simulink library "xrbsImage_r4"  (Simulink 7.1)
libraries: xbsIndex_r4 x24, xrbsDSP_r4 x5, xrbsImage_r4 x4
settings Model: Creator=singhj  LastModifiedBy=sysgengroup

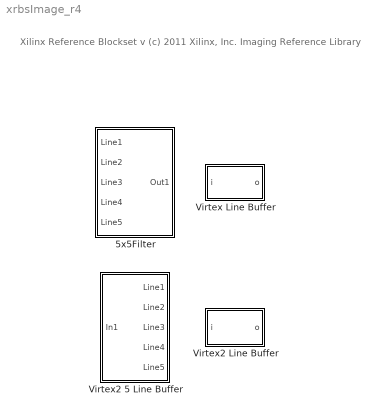
== system xrbsImage_r4 ==
  note: Xilinx Reference Blockset v
      | (c) 2011 Xilinx, Inc.
      |
      | Imaging Reference Library
  5x5Filter : Subsystem  mask(5x5 Filter){maskNum=Edge, coef_n_bits=6, coef_bin_pt=0, smpl_n_bits=8, smpl_bin_pt=0, smpl_period=1, maskVal=0, maskDiv=0}
      mask prompts: maskNum "5x5 Mask"; coef_n_bits "Number of Bits per Coefficient"; coef_bin_pt "Binary Point for Coefficient"; smpl_n_bits "Number of Bits per Input Sample"; smpl_bin_pt "Binary Point for Input Samples"; smpl_period "Sample Period"; maskVal "Mask Value"; maskDiv "Mask Division"
      mask help: The Xilinx 5x5 Filter reference block is implemented using 5 n-tap MAC FIR Filters. Nine different 2-D filters have been provided to filter grayscale images.
      mask init:
      | [bg,fg] = xlcmap('XBlock',0);
      | iPos = get_param(gcb,'Position');
      | iWidth=iPos(3)-iPos(1); iHeight=iPos(4)-iPos(2);
      | iCx=iWidth/2;
      | iCy=iHeight/2;
      | [logoX, logoY] = xlogo(iPos);
      | 
      | % Different 5x5 Filters 
      | %  by default edge is used
      | 
      | edge = [ 0  0  0  0 0; ...
      |          0 -1 -1 -1 0; ...
      |          0 -1  8 -1 0; ...
      |          0 -1 -1 -1 0; ...
      |          0  0  0  0 0];
      | edgeDiv = 1;
      | 
      | sobelX = [ 0  0  0  0 0; ...
      |            0 -1  0  1 0; ...
      |            0 -2  0  2 0; ...
      |            0 -1  0  1 0; ...
      |            0  0  0  0 0];
      | sobelXDiv = 1;
      | 
      | sobelY = [ 0  0  0  0 0; ...
      |            0  1  2  1 0; ...
      |            0  0  0  0 0; ...
      |            0 -1 -2 -1 0; ...
      |            0  0  0  0 0];
      | sobelYDiv = 1;
      | 
      | sobelXY = [ 0  0  0  0 0; ...
      |             0  0 -1 -1 0; ...
      |             0  1  0 -1 0; ...
      |             0  1  1  0 0; ...
      |             0  0  0  0 0];
      | sobelXYDiv = 1;
      | 
      | blur = [ 1  1  1  1 1; ...
      |          1  0  0  0 1; ...
      |          1  0  0  0 1; ...
      |          1  0  0  0 1; ...
      |          1  1  1  1 1];
      | blurDiv = 1/16;
      | 
      | smooth = [ 1  1  1  1 1; ...
      |            1  5  5  5 1; ...
      |            1  5 44  5 1; ...
      |            1  5  5  5 1; ...
      |            1  1  1  1 1];
      | smoothDiv = 1/100;
      | 
      | sharpen = [ 0  0  0  0 0; ...
      |             0 -2 -2 -2 0; ...
      |             0 -2 32 -2 0; ...
      |             0 -2 -2 -2 0; ...
      |             0  0  0  0 0];
      | sharpenDiv = 1/16;
      | 
      | 
      | gaussian = [1 1 2 1 1; ...
      |             1 2 4 2 1; ...
      |             2 4 8 4 2; ...
      |             1 2 4 2 1; ...
      |             1 1 2 1 1];
      | gaussianDiv = 1/52;
      | 
      | identity = [ 0  0  0  0 0; ...
      |              0  0  0  0 0; ...
      |              0  0  1  0 0; ...
      |              0  0  0  0 0; ...
      |              0  0  0  0 0];
      | identityDiv = 1;
      | 
      | maskVal = zeros(5,5,5);
      | maskVal(:,:,1) = edge;
      | maskVal(:,:,2) = sobelX;
      | maskVal(:,:,3) = sobelY;
      | maskVal(:,:,4) = sobelXY;
      | maskVal(:,:,5) = blur;
      | maskVal(:,:,6) = smooth;
      | maskVal(:,:,7) = sharpen;
      | maskVal(:,:,8) = gaussian;
      | maskVal(:,:,9) = identity;
      | 
      | maskDiv = [edgeDiv sobelXDiv sobelYDiv sobelXYDiv blurDiv smoothDiv sharpenDiv gaussianDiv identityDiv];
      mask Help: eval('');xlDoc('-book','sysgen','-topic','x5x5Filter');
      mask StyleString: popup(Edge|Sobel X|Sobel Y|Sobel X-Y|Blur|Smooth|Sharpen|Gaussian|Identity),edit,edit,edit,edit,edit,edit,edit
      mask Display:
      | patch([0 iWidth iWidth 0],[0 0 iHeight iHeight] , bg);
      | patch(logoX,logoY , fg);
      | port_label('input',1,'Line1');
      | port_label('input',2,'Line2');
      | port_label('input',3,'Line3');
      | port_label('input',4,'Line4');
      | port_label('input',5,'Line5');
      | port_label('output',1,'out');
      | plot([0 0 iWidth iWidth 0], [0 iHeight iHeight 0 0]);
  Virtex Line Buffer : Subsystem  mask(Virtex Line Buffer){buf_depth=64, cst=1}
      mask prompts: buf_depth "Buffer Depth"; cst "Sample Period"
      mask help: The Xilinx Virtex Line Buffer reference block delayes a sequential stream of pixels by the specified buffer depth.
      mask init:
      | str = sprintf('-%d',buf_depth);
      | [bg,fg] = xlcmap('XBlock',0);
      | iPos = get_param(gcb,'Position');
      | iWidth=iPos(3)-iPos(1); iHeight=iPos(4)-iPos(2);
      | iCx=iWidth/2;
      | iCy=iHeight/2;
      | [logoX, logoY] = xlogo(iPos);
      mask Help: eval('');xlDoc('-book','sysgen','-topic','Virtex_Line_Buffer');
      mask Display:
      | patch([0 iWidth iWidth 0],[0 0 iHeight iHeight] , bg);
      | patch(logoX,logoY , fg);
      | text(iCx-6,iCy,'z');
      | text(iCx,iCy+4,str);
      | plot([0 0 iWidth iWidth 0], [0 iHeight iHeight 0 0]);
  Virtex2 5 Line Buffer : Subsystem  mask(Virtex2 5 Line Buffer){line_size=64, cst=1}
      mask prompts: line_size "Line Size"; cst "Sample Period"
      mask help: The block buffers a sequential stream of pixels to construct 5 lines of output. Each line is delayed by N samples, where N is the length of the line. Line 1 is delayed 4*N samples, each of the following lines are delay by N fewer samples, and line 5 is a copy of the input.
      mask init:
      | [bg,fg] = xlcmap('XBlock',0);
      | iPos = get_param(gcb,'Position');
      | iWidth=iPos(3)-iPos(1); iHeight=iPos(4)-iPos(2);
      | iCx=iWidth/2;
      | iCy=iHeight/2;
      | [logoX, logoY] = xlogo(iPos);
      mask Help: eval('');xlDoc('-book','sysgen','-topic','Virtex2_5_Line_Buffer');
      mask Display:
      | patch([0 iWidth iWidth 0],[0 0 iHeight iHeight] , bg);
      | patch(logoX,logoY , fg);
      | port_label('input',1,'in');
      | port_label('output',1,'Line1');
      | port_label('output',2,'Line2');
      | port_label('output',3,'Line3');
      | port_label('output',4,'Line4');
      | port_label('output',5,'Line5');
      | plot([0 0 iWidth iWidth 0], [0 iHeight iHeight 0 0]);
  Virtex2 Line Buffer : Subsystem  mask(Virtex2 Line Buffer){buf_depth=64, cst=1}
      mask prompts: buf_depth "Buffer Depth"; cst "Sample Period"
      mask help: The Xilinx Virtex2 Line Buffer reference block delayes a sequential stream of pixels by the specified buffer depth. It is optimized for the Virtex2 family since it uses the Read Before Write option on the underlying Single Port RAM block.
      mask init: same as xrbsImage_r4/Virtex Line Buffer
      mask Help: eval('');xlDoc('-book','sysgen','-topic','Virtex2_Line_Buffer');
      mask Display:
      | patch([0 iWidth iWidth 0],[0 0 iHeight iHeight] , bg);
      | patch(logoX,logoY , fg);
      | text(iCx-6,iCy,'z');
      | text(iCx,iCy+4,str);
      | plot([0 0 iWidth iWidth 0], [0 iHeight iHeight 0 0]);

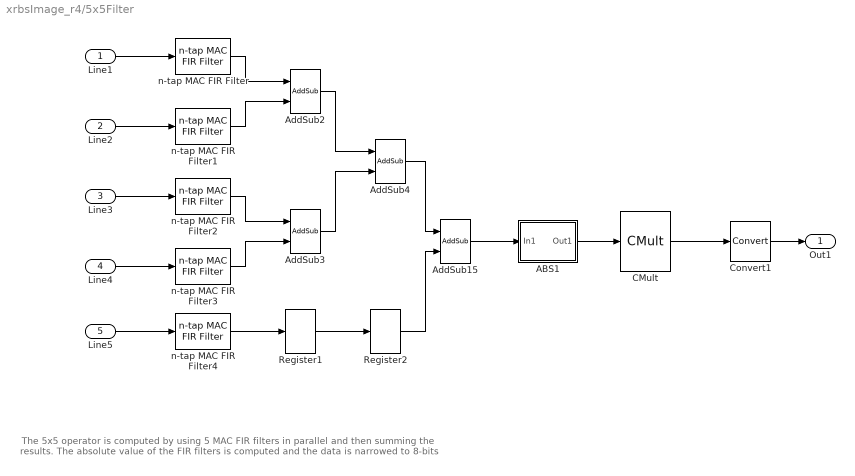
== system xrbsImage_r4/5x5Filter ==
  note: The 5x5 operator is computed by using 5 MAC FIR filters in parallel and then
      | summing the results.  The absolute value of the FIR filters is computed
      | and the data is narrowed to 8-bits
  Line1 : Inport  OutDataType=sfix(16)  OutScaling=2^0
  Line2 : Inport  Port=2  OutDataType=sfix(16)  OutScaling=2^0
  Line3 : Inport  Port=3  OutDataType=sfix(16)  OutScaling=2^0
  Line4 : Inport  Port=4  OutDataType=sfix(16)  OutScaling=2^0
  Line5 : Inport  Port=5  OutDataType=sfix(16)  OutScaling=2^0
  ABS1 : Subsystem
  AddSub{2..4,15} (4 alike) : xbsIndex_r4/AddSub  mode=Addition  use_carryin=off  use_carryout=off  en=off  latency=1  precision=Full  arith_type=Unsigned  n_bits=8  bin_pt=2  quantization=Truncate  overflow=Wrap  dbl_ovrd=off  use_behavioral_HDL=off  pipelined=off  use_rpm=off  block_type=addsub
      settings: xl_area=[0, 0, 0, 0, 0, 0, 0]  block_version=VER_STRING_GOES_HERE
  CMult : xbsIndex_r4/CMult  const=maskDiv(maskNum)  const_n_bits=18  const_bin_pt=17  en=off  latency=4  precision=Full  arith_type=Unsigned  n_bits=8  bin_pt=0  quantization=Truncate  overflow=Wrap  dbl_ovrd=off  use_behavioral_HDL=off  mem_type=Distributed RAM  placement_style=Rectangular Shape  pipeline=on  use_rpm=off  block_type=cmult
      settings: xl_area=[0, 0, 0, 0, 0, 0, 0]  infoedit="Hardware notes: The hardware oversampling rate determines the degree of parallelism in the constant sequential multiplier.  A rate of n for n-bit input signals produces a fully serial implementation.  Intermediate values produce implementations with intermediate levels of parallelism."  block_version=VER_STRING_GOES_HERE
  Convert1 : xbsIndex_r4/Convert  arith_type=Unsigned  n_bits=8  bin_pt=0  quantization=Truncate  overflow=Saturate  latency=1  dbl_ovrd=off  pipeline=off  block_type=convert
      settings: infoedit=The input is presented at the output after quantization and overflow effects.<P><P>Hardware notes: Additional hardware is used when rounding or saturation is selected and output width is less than the input width.  xl_area=[0, 0, 0, 0, 0, 0, 0]  block_version=VER_STRING_GOES_HERE
  Register1 : xbsIndex_r4/Register  init=0  rst=off  en=off  dbl_ovrd=off  block_type=register
      settings: xl_area=[0, 0, 0, 0, 0, 0, 0]  block_version=VER_STRING_GOES_HERE
  Register2 : xbsIndex_r4/Register  init=0  rst=off  en=off  dbl_ovrd=off  block_type=register
      settings: xl_area=[0, 0, 0, 0, 0, 0, 0]  block_version=VER_STRING_GOES_HERE
  n-tap MAC FIR Filter : xrbsDSP_r4/n-tap MAC FIR Filter  SystemSampleTime=-1  coef=maskVal(1,5:-1:1,maskNum)  coef_n_bits=coef_n_bits  coef_bin_pt=coef_bin_pt  smpl_n_bits=smpl_n_bits  smpl_bin_pt=smpl_bin_pt  smpl_period=smpl_period
  n-tap MAC FIR Filter1 : xrbsDSP_r4/n-tap MAC FIR Filter  SystemSampleTime=-1  coef=maskVal(2,5:-1:1,maskNum)  coef_n_bits=coef_n_bits  coef_bin_pt=coef_bin_pt  smpl_n_bits=smpl_n_bits  smpl_bin_pt=smpl_bin_pt  smpl_period=smpl_period
  n-tap MAC FIR Filter2 : xrbsDSP_r4/n-tap MAC FIR Filter  SystemSampleTime=-1  coef=maskVal(3,5:-1:1,maskNum)  coef_n_bits=coef_n_bits  coef_bin_pt=coef_bin_pt  smpl_n_bits=smpl_n_bits  smpl_bin_pt=smpl_bin_pt  smpl_period=smpl_period
  n-tap MAC FIR Filter3 : xrbsDSP_r4/n-tap MAC FIR Filter  SystemSampleTime=-1  coef=maskVal(4,5:-1:1,maskNum)  coef_n_bits=coef_n_bits  coef_bin_pt=coef_bin_pt  smpl_n_bits=smpl_n_bits  smpl_bin_pt=smpl_bin_pt  smpl_period=smpl_period
  n-tap MAC FIR Filter4 : xrbsDSP_r4/n-tap MAC FIR Filter  SystemSampleTime=-1  coef=maskVal(5,5:-1:1,maskNum)  coef_n_bits=coef_n_bits  coef_bin_pt=coef_bin_pt  smpl_n_bits=smpl_n_bits  smpl_bin_pt=smpl_bin_pt  smpl_period=smpl_period
  Out1 : Outport  OutDataType=sfix(16)  OutScaling=2^0
  wires:
  Line1/1 -> n-tap MAC FIR Filter/1
  Line2/1 -> n-tap MAC FIR Filter1/1
  Line3/1 -> n-tap MAC FIR Filter2/1
  Line4/1 -> n-tap MAC FIR Filter3/1
  Line5/1 -> n-tap MAC FIR Filter4/1
  n-tap MAC FIR Filter/1 -> AddSub2/1
  n-tap MAC FIR Filter1/1 -> AddSub2/2
  n-tap MAC FIR Filter2/1 -> AddSub3/1
  n-tap MAC FIR Filter3/1 -> AddSub3/2
  AddSub2/1 -> AddSub4/1
  AddSub3/1 -> AddSub4/2
  n-tap MAC FIR Filter4/1 -> Register1/1
  Register1/1 -> Register2/1
  AddSub15/1 -> ABS1/1(In1)
  AddSub4/1 -> AddSub15/1
  Register2/1 -> AddSub15/2
  CMult/1 -> Convert1/1
  ABS1/1(Out1) -> CMult/1
  Convert1/1 -> Out1/1

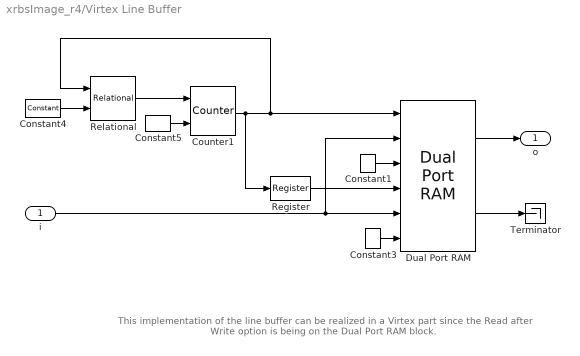
== system xrbsImage_r4/Virtex Line Buffer ==
  note: This implementation of the line buffer can be realized in a Virtex
      | part since the Read after Write option is being on the
      |  Dual Port RAM block.
  i : Inport  OutDataType=sfix(16)  OutScaling=2^0
  Constant1 : xbsIndex_r4/Constant  arith_type=Boolean  const=0  n_bits=1  bin_pt=0  explicit_period=off  period=cst  equ=P=C  opselect=C  inp2=PCIN>>17  opr=+  inp1=P  carry=CIN  dbl_ovrd=off  block_type=constant
      settings: block_version=VER_STRING_GOES_HERE
  Constant3 : xbsIndex_r4/Constant  arith_type=Boolean  const=1  n_bits=1  bin_pt=0  explicit_period=off  period=cst  equ=P=C  opselect=C  inp2=PCIN>>17  opr=+  inp1=P  carry=CIN  dbl_ovrd=off  block_type=constant
      settings: block_version=VER_STRING_GOES_HERE
  Constant4 : xbsIndex_r4/Constant  arith_type=Unsigned  const=buf_depth-1  n_bits=ceil(log2(buf_depth))  bin_pt=0  explicit_period=off  period=cst  equ=P=C  opselect=C  inp2=PCIN>>17  opr=+  inp1=P  carry=CIN  dbl_ovrd=off  block_type=constant
      settings: block_version=VER_STRING_GOES_HERE
  Constant5 : xbsIndex_r4/Constant  arith_type=Unsigned  const=0  n_bits=ceil(log2(buf_depth))  bin_pt=0  explicit_period=on  period=cst  equ=P=C  opselect=C  inp2=PCIN>>17  opr=+  inp1=P  carry=CIN  dbl_ovrd=off  block_type=constant
      settings: block_version=VER_STRING_GOES_HERE
  Counter1 : xbsIndex_r4/Counter  cnt_type=Free Running  cnt_to=buf_depth -1  operation=Up  start_count=1  cnt_by_val=1  arith_type=Unsigned  n_bits=ceil(log2(buf_depth))  bin_pt=0  load_pin=on  rst=off  en=off  dbl_ovrd=off  explicit_period=off  period=cst  block_type=counter
      settings: infoedit="Configurable up, down and up/down counter.<P><P>Hardware notes: Free running counters are the least expensive in hardware.  A count limited counter is implemented by combining a counter with a comparator."  xl_area=[6 10 0 11 0 0 0]  block_version=VER_STRING_GOES_HERE
  Dual Port RAM : xbsIndex_r4/Dual Port RAM  depth=buf_depth  initVector=0  distributed_mem=Block RAM  init_a=0  init_b=0  rst_a=off  rst_b=off  en_a=off  en_b=off  latency=1  write_mode_A=Read After Write  write_mode_B=Read After Write  dbl_ovrd=off  explicit_period=off  period=-1  use_rpm=off  block_type=dpram
      settings: infoedit=Independent address, data and write enable ports allow shared access to a single memory space. Dual ports enable simultaneous access to the memory space at different sample rates using multiple data widths.  xl_area=[0 0 1 0 0 0 0]  block_version=VER_STRING_GOES_HERE
  Register : xbsIndex_r4/Register  init=0  rst=off  en=off  dbl_ovrd=off  block_type=register
      settings: infoedit=Delay of one sample period. <P><P>Hardware notes: Implemented using flip-flops.  xl_area=[5 10 0 0 0 0 0]  block_version=VER_STRING_GOES_HERE
  Relational : xbsIndex_r4/Relational  mode=a=b  en=off  latency=0  dbl_ovrd=off  block_type=relational
      settings: xl_area=[4 0 0 3 0 0 0]  block_version=VER_STRING_GOES_HERE
  Terminator : Terminator
  o : Outport  OutDataType=sfix(16)  OutScaling=2^0
  wires:
  Dual Port RAM/2 -> Terminator/1
  i/1 -> Dual Port RAM/5, Dual Port RAM/2
  Dual Port RAM/1 -> o/1
  Constant3/1 -> Dual Port RAM/6
  Constant1/1 -> Dual Port RAM/3
  Counter1/1 -> Relational/1, Dual Port RAM/1, Register/1
  Relational/1 -> Counter1/1
  Constant4/1 -> Relational/2
  Register/1 -> Dual Port RAM/4
  Constant5/1 -> Counter1/2

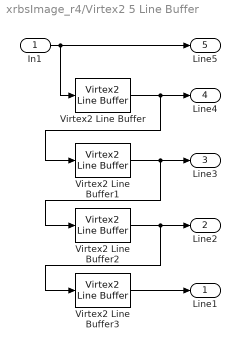
== system xrbsImage_r4/Virtex2 5 Line Buffer ==
  In1 : Inport  OutDataType=sfix(16)  OutScaling=2^0
  Virtex2 Line Buffer{,1..3} (4 alike) : xrbsImage_r4/Virtex2 Line Buffer  buf_depth=line_size  cst=cst
  Line1 : Outport  OutDataType=sfix(16)  OutScaling=2^0
  Line2 : Outport  Port=2  OutDataType=sfix(16)  OutScaling=2^0
  Line3 : Outport  Port=3  OutDataType=sfix(16)  OutScaling=2^0
  Line4 : Outport  Port=4  OutDataType=sfix(16)  OutScaling=2^0
  Line5 : Outport  Port=5  OutDataType=sfix(16)  OutScaling=2^0
  wires:
  In1/1 -> Line5/1, Virtex2 Line Buffer/1
  Virtex2 Line Buffer/1 -> Line4/1, Virtex2 Line Buffer1/1
  Virtex2 Line Buffer1/1 -> Line3/1, Virtex2 Line Buffer2/1
  Virtex2 Line Buffer2/1 -> Line2/1, Virtex2 Line Buffer3/1
  Virtex2 Line Buffer3/1 -> Line1/1

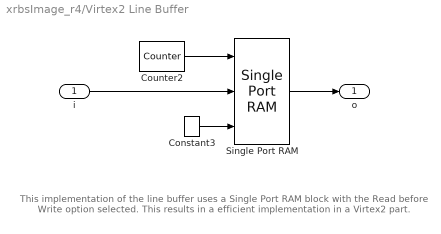
== system xrbsImage_r4/Virtex2 Line Buffer ==
  note: This implementation of the line buffer uses a
      |  Single Port RAM block with the Read before Write
      | option selected.  This results in a efficient
      | implementation in a Virtex2 part.
  i : Inport  OutDataType=sfix(16)  OutScaling=2^0
  Constant3 : xbsIndex_r4/Constant  arith_type=Boolean  const=1  n_bits=1  bin_pt=0  explicit_period=on  period=cst  equ=P=C  opselect=C  inp2=PCIN>>17  opr=+  inp1=P  carry=CIN  dbl_ovrd=off  block_type=constant
      settings: block_version=VER_STRING_GOES_HERE
  Counter2 : xbsIndex_r4/Counter  cnt_type=Count Limited  cnt_to=buf_depth -2  operation=Up  start_count=0  cnt_by_val=1  arith_type=Unsigned  n_bits=ceil(log2(buf_depth-1))  bin_pt=0  load_pin=off  rst=off  en=off  dbl_ovrd=off  explicit_period=on  period=cst  block_type=counter
      settings: infoedit="Configurable up, down and up/down counter.<P><P>Hardware notes: Free running counters are the least expensive in hardware.  A count limited counter is implemented by combining a counter with a comparator."  xl_area=[7 10 0 13 0 0 0]  block_version=VER_STRING_GOES_HERE
  Single Port RAM : xbsIndex_r4/Single Port RAM  depth=buf_depth-1  initVector=0  write_mode=Read Before Write  rst=off  init_reg=0  en=off  latency=1  dbl_ovrd=off  distributed_mem=Block RAM  use_rpm=off  block_type=spram
      settings: xl_area=[0 0 1 0 0 0 0]  block_version=VER_STRING_GOES_HERE
  o : Outport  OutDataType=sfix(16)  OutScaling=2^0
  wires:
  Constant3/1 -> Single Port RAM/3
  Single Port RAM/1 -> o/1
  i/1 -> Single Port RAM/2
  Counter2/1 -> Single Port RAM/1

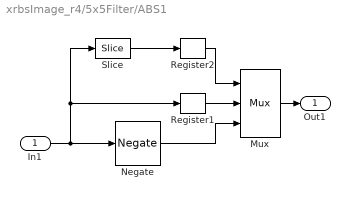
== system xrbsImage_r4/5x5Filter/ABS1 ==
  In1 : Inport  OutDataType=sfix(16)  OutScaling=2^0
  Mux : xbsIndex_r4/Mux  inputs=2  en=off  latency=1  precision=Full  arith_type=Unsigned  n_bits=8  bin_pt=0  quantization=Truncate  overflow=Saturate  dbl_ovrd=off  block_type=mux
      settings: xl_area=[0, 0, 0, 0, 0, 0, 0]  infoedit=Binary points are aligned automatically.<P><P>Hardware notes: A multiplexer using tristate buffers requires fewer lookup tables but is slower.  block_version=VER_STRING_GOES_HERE
  Negate : xbsIndex_r4/Negate  precision=Full  arith_type=Unsigned  n_bits=8  bin_pt=2  quantization=Truncate  overflow=Wrap  en=off  latency=1  dbl_ovrd=off  block_type=negate
      settings: xl_area=[0, 0, 0, 0, 0, 0, 0]  block_version=VER_STRING_GOES_HERE
  Register1 : xbsIndex_r4/Register  init=0  rst=off  en=off  dbl_ovrd=off  block_type=register
      settings: xl_area=[0, 0, 0, 0, 0, 0, 0]  block_version=VER_STRING_GOES_HERE
  Register2 : xbsIndex_r4/Register  init=0  rst=off  en=off  dbl_ovrd=off  block_type=register
      settings: xl_area=[0, 0, 0, 0, 0, 0, 0]  block_version=VER_STRING_GOES_HERE
  Slice : xbsIndex_r4/Slice  nbits=1  boolean_output=off  mode=Upper Bit Location + Width  bit1=0  base1=MSB of Input  bit0=0  base0=LSB of Input  dbl_ovrd=off  block_type=slice
      settings: infoedit="Extracts a given range of bits from each input sample and presents it at the output.  The output type is ordinarily unsigned with binary point at zero, but can be Boolean when the slice is one bit wide.<P><P>Hardware notes: In hardware this block costs nothing."  block_version=VER_STRING_GOES_HERE
  Out1 : Outport  OutDataType=sfix(16)  OutScaling=2^0
  wires:
  Register1/1 -> Mux/2
  Register2/1 -> Mux/1
  Mux/1 -> Out1/1
  In1/1 -> Register1/1, Slice/1, Negate/1
  Negate/1 -> Mux/3
  Slice/1 -> Register2/1
